simulink model "today4Zapazdavanie"  (R2016a)
settings: Solver=VariableStepAuto  StartTime=0.0  StopTime=10.0  RelTol=1e-3
settings Model: Creator=Ivan Varabei  LastModifiedBy=Ivan Varabei

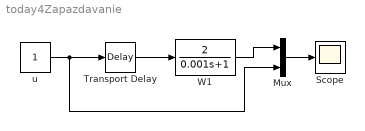
== system today4Zapazdavanie ==
  Mux : Mux  Inputs=2
  Scope : Scope
  Transport Delay : TransportDelay  DelayTime=6.8
  "W1 " : TransferFcn  Numerator=[2]  Denominator=[0.001 1]
  u : Constant
  wires:
  Transport Delay/1 -> "W1 "/1
  u/1 -> Mux/2, Transport Delay/1
  Mux/1 -> Scope/1
  "W1 "/1 -> Mux/1
